simulink model "flight_sim"  (R2018b)
settings: Solver=FixedStepAuto  StartTime=0.0  StopTime=10  FixedStep=1.5  RelTol=1e-3
libraries: simulink x2, simulink_extras x1
settings Model: Creator=User  LastModifiedBy=Танечка
settings DebuggingCC: LibraryContextMissingDiagnostic=none
settings SFSimCC: SimUseLocalCustomCode=off
settings RTWCC: RTWUseLocalCustomCode=off

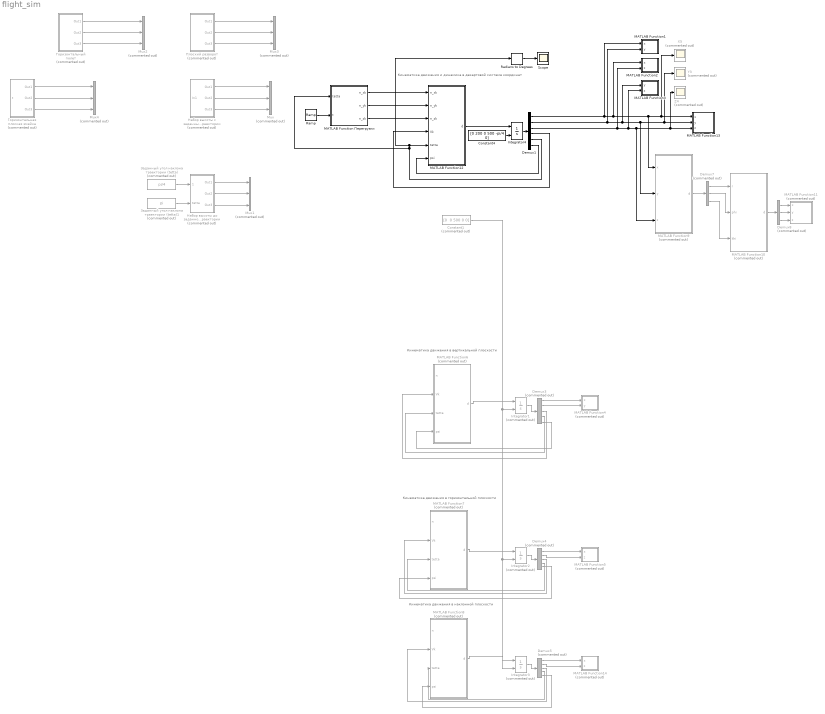
== system flight_sim ==
  note: Кинематика движения и динамика в декартовой системе координат
  note: Кинематика движения в вертикальной плоскости
  note: Кинематика движения в горизонтальной плоскости
  note: Кинематика движения в наклонной плоскости
  Constant1 : Constant  Commented=on  Value="[0  0 500 0 0]"
  Constant4 : Constant  Value=[0 200 0 500 -pi/4 0]
  Demux1 : Demux  Outputs=6
  Demux3 : Demux  Commented=on  Outputs=5
  Demux4 : Demux  Commented=on  Outputs=5
  Demux5 : Demux  Commented=on  Outputs=5
  Demux7 : Demux  Commented=on  Outputs=3
  Demux8 : Demux  Commented=on  Outputs=3
  Integrator1 : Integrator  Commented=on  InitialConditionSource=external
  Integrator2 : Integrator  Commented=on  InitialConditionSource=external
  Integrator3 : Integrator  Commented=on  InitialConditionSource=external
  Integrator4 : Integrator  InitialConditionSource=external
  MATLAB Function Перегрузки : MATLAB Function  TreatAsAtomicUnit=on
  MATLAB Function1 : MATLAB Function  TreatAsAtomicUnit=on
  MATLAB Function10 : MATLAB Function  Commented=on  TreatAsAtomicUnit=on
  MATLAB Function11 : MATLAB Function  Commented=on  TreatAsAtomicUnit=on
  MATLAB Function12 : MATLAB Function  TreatAsAtomicUnit=on
  MATLAB Function13 : MATLAB Function  TreatAsAtomicUnit=on
  MATLAB Function14 : MATLAB Function  Commented=on  TreatAsAtomicUnit=on
  MATLAB Function2 : MATLAB Function  TreatAsAtomicUnit=on
  MATLAB Function3 : MATLAB Function  TreatAsAtomicUnit=on
  MATLAB Function4 : MATLAB Function  Commented=on  TreatAsAtomicUnit=on
  MATLAB Function5 : MATLAB Function  Commented=on  TreatAsAtomicUnit=on
  MATLAB Function6 : MATLAB Function  Commented=on  TreatAsAtomicUnit=on
  MATLAB Function7 : MATLAB Function  Commented=on  TreatAsAtomicUnit=on
  MATLAB Function8 : MATLAB Function  Commented=on  TreatAsAtomicUnit=on
  MATLAB Function9 : MATLAB Function  Commented=on  TreatAsAtomicUnit=on
  Mux{,1..4} (5 alike) : Mux  Commented=on  Inputs=3
  Radians to Degrees : simulink_extras/Transformations/Radians to Degrees
  Ramp : simulink/Sources/Ramp  slope=1  start=0  InitialOutput=0
  Scope : Scope
  X5 : Scope  Commented=on
  Y3 : Scope  Commented=on
  Z4 : Scope  Commented=on
  Горизонтальная плоская змейка : Subsystem  Commented=on
  Горизонтальный полет : Subsystem  Commented=on
  Заданный угол наклона траектории (tetta) : Constant  Commented=on  Value=pi/4
  Заданный угол наклона траектории (tetta)1 : Constant  Commented=on  Value=pi
  Набор высоты до заданного угла наклона траектории : Subsystem  Commented=on
  "Набор высоты с заданным углом наклона траектории " : Subsystem  Commented=on
  Плоский разворот : Subsystem  Commented=on
  wires:
  Demux1/3 -> MATLAB Function2/2(z), MATLAB Function3/2(z), MATLAB Function9/3(z), MATLAB Function13/3(z), Z4/1
  Demux7/3 -> MATLAB Function10/3(khi)
  Demux7/2 -> MATLAB Function10/2(phi)
  Demux1/1 -> MATLAB Function1/1(x), MATLAB Function2/1(x), MATLAB Function9/1(x), X5/1, MATLAB Function13/1(x)
  Constant4/1 -> Integrator4/2
  MATLAB Function9/1(d) -> Demux7/1
  Demux1/5 -> MATLAB Function Перегрузки/1(tetta), MATLAB Function12/5(tetta), Radians to Degrees/1
  MATLAB Function10/1(d) -> Demux8/1
  Demux1/4 -> MATLAB Function12/4(Vk)
  Demux7/1 -> MATLAB Function10/1(r)
  Demux1/6 -> MATLAB Function12/6(psi)
  Integrator3/1 -> Demux5/1
  Demux3/2 -> MATLAB Function4/2(y)
  Constant1/1 -> Integrator1/2, Integrator3/2, Integrator2/2
  Integrator1/1 -> Demux3/1
  Demux5/2 -> MATLAB Function14/2(z)
  MATLAB Function6/1(d) -> Integrator1/1
  MATLAB Function8/1(d) -> Integrator3/1
  Demux5/1 -> MATLAB Function14/1(x)
  Demux4/2 -> MATLAB Function5/2(z)
  MATLAB Function7/1(d) -> Integrator2/1
  Integrator2/1 -> Demux4/1
  Demux4/1 -> MATLAB Function5/1(x)
  Demux3/1 -> MATLAB Function4/1(x)
  Demux3/3 -> MATLAB Function6/2(Vk)
  Demux3/4 -> MATLAB Function6/3(tetta)
  Demux3/5 -> MATLAB Function6/4(psi)
  Demux4/3 -> MATLAB Function7/2(Vk)
  Demux4/4 -> MATLAB Function7/3(tetta)
  Demux4/5 -> MATLAB Function7/4(psi)
  Demux5/3 -> MATLAB Function8/2(Vk)
  Demux5/4 -> MATLAB Function8/3(tetta)
  Demux5/5 -> MATLAB Function8/4(psi)
  Demux8/1 -> MATLAB Function11/1(x)
  Demux8/2 -> MATLAB Function11/2(y)
  Demux8/3 -> MATLAB Function11/3(z)
  MATLAB Function12/1(d) -> Integrator4/1
  Integrator4/1 -> Demux1/1
  Demux1/2 -> MATLAB Function1/2(y), MATLAB Function3/1(y), Y3/1, MATLAB Function13/2(y), MATLAB Function9/2(y)
  "Набор высоты с заданным углом наклона траектории "/1(Out1) -> Mux/1
  "Набор высоты с заданным углом наклона траектории "/2(Out2) -> Mux/2
  "Набор высоты с заданным углом наклона траектории "/3(Out3) -> Mux/3
  Заданный угол наклона траектории (tetta)/1 -> Набор высоты до заданного угла наклона траектории/1(tetta заданноне)
  Набор высоты до заданного угла наклона траектории/1(Out1) -> Mux1/1
  Набор высоты до заданного угла наклона траектории/2(Out2) -> Mux1/2
  Набор высоты до заданного угла наклона траектории/3(Out3) -> Mux1/3
  Заданный угол наклона траектории (tetta)1/1 -> Набор высоты до заданного угла наклона траектории/2(tetta)
  Горизонтальный полет/3(Out3) -> Mux2/3
  Горизонтальный полет/2(Out2) -> Mux2/2
  Горизонтальный полет/1(Out1) -> Mux2/1
  Плоский разворот/1(Out1) -> Mux3/1
  Плоский разворот/2(Out2) -> Mux3/2
  Плоский разворот/3(Out3) -> Mux3/3
  Горизонтальная плоская змейка/3(Out3) -> Mux4/3
  Горизонтальная плоская змейка/2(Out2) -> Mux4/2
  Горизонтальная плоская змейка/1(Out1) -> Mux4/1
  MATLAB Function Перегрузки/1(n_xk) -> MATLAB Function12/1(n_xk)
  MATLAB Function Перегрузки/2(n_yk) -> MATLAB Function12/2(n_yk)
  MATLAB Function Перегрузки/3(n_zk) -> MATLAB Function12/3(n_zk)
  Ramp/1 -> MATLAB Function Перегрузки/2(t)
  Radians to Degrees/1 -> Scope/1

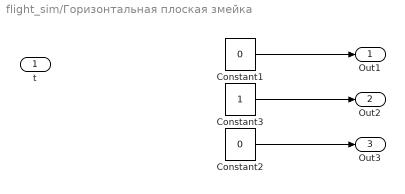
== system flight_sim/Горизонтальная плоская змейка ==
  t : Inport
  Constant1 : Constant  Value=0
  Constant2 : Constant  Value=0
  Constant3 : Constant
  Out1 : Outport
  Out2 : Outport  Port=2
  Out3 : Outport  Port=3
  wires:
  Constant2/1 -> Out3/1
  Constant3/1 -> Out2/1
  Constant1/1 -> Out1/1

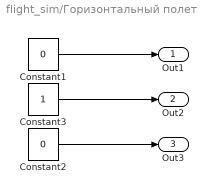
== system flight_sim/Горизонтальный полет ==
  Constant1 : Constant  Value=0
  Constant2 : Constant  Value=0
  Constant3 : Constant
  Out1 : Outport
  Out2 : Outport  Port=2
  Out3 : Outport  Port=3
  wires:
  Constant2/1 -> Out3/1
  Constant3/1 -> Out2/1
  Constant1/1 -> Out1/1

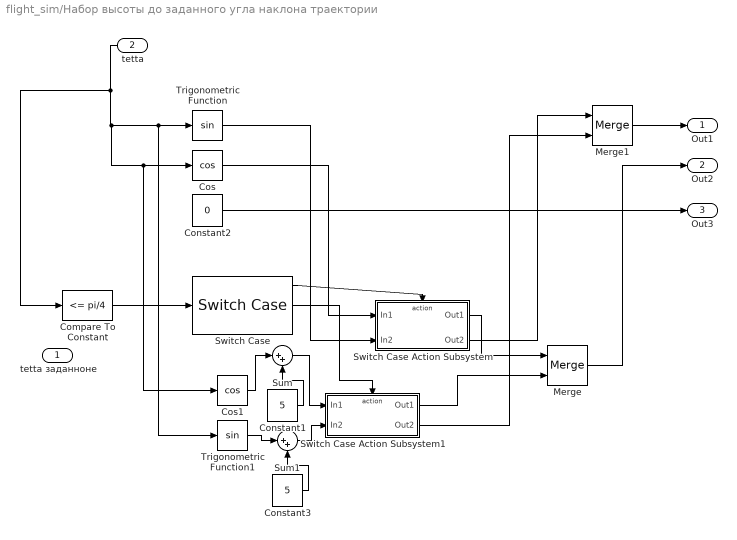
== system flight_sim/Набор высоты до заданного угла наклона траектории ==
  tetta заданноне : Inport
  tetta : Inport  Port=2
  Compare To Constant : simulink/Logic and Bit Operations/Compare To Constant  relop=<=  const=pi/4  OutDataTypeStr=uint8
  Constant1 : Constant  Value=5
  Constant2 : Constant  Value=0
  Constant3 : Constant  Value=5
  Cos : Trigonometry  Operator=cos
  Cos1 : Trigonometry  Operator=cos
  Merge : Merge
  Merge1 : Merge
  Sum : Sum  Inputs=|++
  Sum1 : Sum  Inputs=|++
  Switch Case : SwitchCase  CaseConditions={0,1}
  Switch Case Action Subsystem : Subsystem  TreatAsAtomicUnit=on
  Switch Case Action Subsystem1 : Subsystem  TreatAsAtomicUnit=on
  Trigonometric Function : Trigonometry
  Trigonometric Function1 : Trigonometry
  Out1 : Outport
  Out2 : Outport  Port=2
  Out3 : Outport  Port=3
  wires:
  Constant2/1 -> Out3/1
  Switch Case/1 -> Switch Case Action Subsystem/Action
  Switch Case/2 -> Switch Case Action Subsystem1/Action
  Switch Case Action Subsystem/1(Out1) -> Merge/1
  Switch Case Action Subsystem1/1(Out1) -> Merge/2
  Merge/1 -> Out2/1
  Cos/1 -> Switch Case Action Subsystem/1(In1)
  Cos1/1 -> Sum/1
  Compare To Constant/1 -> Switch Case/1
  Merge1/1 -> Out1/1
  Switch Case Action Subsystem/2(Out2) -> Merge1/1
  Switch Case Action Subsystem1/2(Out2) -> Merge1/2
  Trigonometric Function/1 -> Switch Case Action Subsystem/2(In2)
  tetta/1 -> Trigonometric Function1/1, Trigonometric Function/1, Cos/1, Cos1/1, Compare To Constant/1
  Sum/1 -> Switch Case Action Subsystem1/1(In1)
  Constant1/1 -> Sum/2
  Constant3/1 -> Sum1/2
  Trigonometric Function1/1 -> Sum1/1
  Sum1/1 -> Switch Case Action Subsystem1/2(In2)

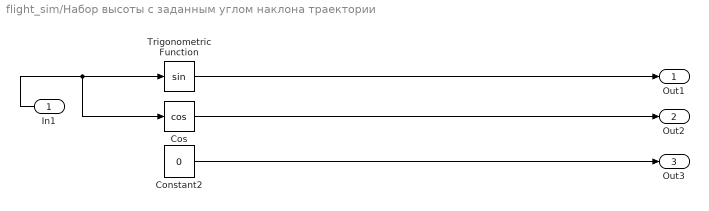
== system flight_sim/Набор высоты с заданным углом наклона траектории  ==
  In1 : Inport
  Constant2 : Constant  Value=0
  Cos : Trigonometry  Operator=cos
  Trigonometric Function : Trigonometry
  Out1 : Outport
  Out2 : Outport  Port=2
  Out3 : Outport  Port=3
  wires:
  Cos/1 -> Out2/1
  Constant2/1 -> Out3/1
  Trigonometric Function/1 -> Out1/1
  In1/1 -> Trigonometric Function/1, Cos/1

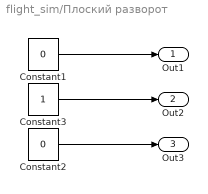
== system flight_sim/Плоский разворот ==
  Constant1 : Constant  Value=0
  Constant2 : Constant  Value=0
  Constant3 : Constant
  Out1 : Outport
  Out2 : Outport  Port=2
  Out3 : Outport  Port=3
  wires:
  Constant1/1 -> Out1/1
  Constant3/1 -> Out2/1
  Constant2/1 -> Out3/1

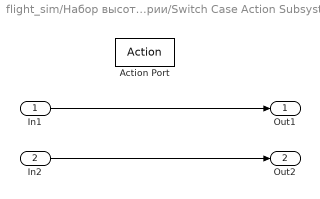
== system flight_sim/Набор высоты до заданного угла наклона траектории/Switch Case Action Subsystem ==
  In1 : Inport
  In2 : Inport  Port=2
  Action Port : ActionPort  ActionType=case
  Out1 : Outport
  Out2 : Outport  Port=2
  wires:
  In1/1 -> Out1/1
  In2/1 -> Out2/1

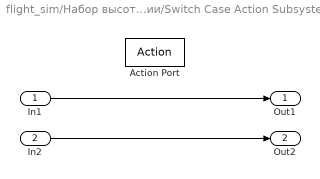
== system flight_sim/Набор высоты до заданного угла наклона траектории/Switch Case Action Subsystem1 ==
  In1 : Inport
  In2 : Inport  Port=2
  Action Port : ActionPort  ActionType=case
  Out1 : Outport
  Out2 : Outport  Port=2
  wires:
  In1/1 -> Out1/1
  In2/1 -> Out2/1

== matlab function flight_sim/MATLAB Function1 ==
  data: x input; y input
function plot2d(x,y)

figure(1);
plot(x,y,'ob');
hold on;

grid on;

xlabel('X');
ylabel('Y');
end

== matlab function flight_sim/MATLAB Function2 ==
  data: x input; z input
function plot2d(x,z)

figure(2);
plot(x,z,'ob');
hold on;

grid on;
xlabel('X');
ylabel('Z');
end

== matlab function flight_sim/MATLAB Function3 ==
  data: y input; z input
function plot2d(y,z)

figure(3);
plot(y,z,'ob');
hold on;

grid on;
xlabel('Y');
ylabel('Z');
end

== matlab function flight_sim/MATLAB Function6 ==
  data: n input; Vk input; d output; tetta input; psi input
function d  = diff(n,Vk,tetta,psi)

g = 9.81;
n_xk = n(1);
n_yk = n(2);
n_zk = n(3);

% Траекторного движения в вертикальной плоскости

dxg = Vk*cos(tetta)*cos(psi);      %xg
dyg = Vk*sin(tetta);               %yg

% Динамика траекторного движения
dVk    = g*(n_xk - sin(tetta));
dtetta = (g/Vk)*(n_yk - cos(tetta));
dpsi   = -(g*n_zk)/(Vk*cos(tetta));

d = [dxg dyg dVk dtetta dpsi];

end

== matlab function flight_sim/MATLAB Function14 ==
  data: x input; z input
function plot2d(x,z)

figure(7);
plot(x,z,'ob');
hold on;

grid on;
title('Движение в наклонной плоскости');
xlabel('X');
ylabel('Z');
end

== matlab function flight_sim/MATLAB Function4 ==
  data: x input; y input
function plot2d(x,y)

figure(5);
plot(x,y,'ob');
hold on;

grid on;
title('Движение в вертикальной плоскости');
xlabel('X');
ylabel('Y');
end

== matlab function flight_sim/MATLAB Function7 ==
  data: n input; Vk input; d output; tetta input; psi input
function d  = diff(n, Vk,tetta,psi)

g = 9.81;
n_xk = n(1);
n_yk = n(2);
n_zk = n(3);

% Траекторного движения в горизонтальной плоскости

dxg = Vk*cos(tetta)*cos(psi);      %xg
dzg = -Vk*cos(tetta)*sin(psi);     %zg

% Динамика траекторного движения
dVk    = g*(n_xk - sin(tetta));
dtetta = (g/Vk)*(n_yk - cos(tetta));
dpsi   = -(g*n_zk)/(Vk*cos(tetta));

d = [dxg dzg dVk dtetta dpsi];

end

== matlab function flight_sim/MATLAB Function8 ==
  data: n input; Vk input; d output; tetta input; psi input
function d  = diff(n, Vk,tetta,psi)

g = 9.81;
n_xk = n(1);
n_yk = n(2);
n_zk = n(3);


% Траекторного движения в наклонная плоскости

dxg = Vk*cos(psi);     %xg
dzg = -Vk*sin(psi);    %zg

% Динамика траекторного движения
dVk    = g*(n_xk - sin(tetta));
dtetta = (g/Vk)*(n_yk - cos(tetta));
dpsi   = -(g*n_zk)/(Vk*cos(tetta));

d = [dxg dzg dVk dtetta dpsi];
end

== matlab function flight_sim/MATLAB Function10 ==
  data: r input; d output; phi input; khi input
function d  = diff(r, phi, khi)

% Из сферической системе координат в декартову

dx = r*cos(phi)*cos(khi);
dy = r*sin(phi);             
dz = -r*cos(phi)*sin(khi);     

d = [dx dy dz];

end

== matlab function flight_sim/MATLAB Function11 ==
  data: x input; y input; z input
function plot3d(x,y, z)

figure(2);
plot3(x,z,y,'ob');
hold on;

grid on;

end

== matlab function flight_sim/MATLAB Function12 ==
  data: n_xk input; n_yk input; n_zk input; Vk input; d output; tetta input; psi input
function d  = diff(n_xk, n_yk, n_zk, Vk,tetta,psi)

% n_xk = n(1);
% n_yk = n(2);
% n_zk = n(3);

% tetta = deg2rad(tetta);
% psi   = deg2rad(psi);
g = 9.81;

% Кинематика траекторного движения
dxg = Vk*cos(tetta)*cos(psi);      %xg
dyg = Vk*sin(tetta);               %yg
dzg = -Vk*cos(tetta)*sin(psi);     %zg


% % Динамика траекторного движения
dVk    = g*(n_xk - sin(tetta));
dtetta = (g/Vk)*(n_yk - cos(tetta));
dpsi   = -(g*n_zk)/(Vk*cos(tetta));

d = [dxg dyg dzg dVk dtetta dpsi];
end

== matlab function flight_sim/MATLAB Function13 ==
  data: x input; y input; z input
function plot3d(x,y, z)

figure(4);
plot3(x,z,y,'ob');
hold on;

grid on;
xlabel('X');
ylabel('Z');
zlabel('Y');

end

== matlab function flight_sim/MATLAB Function9 ==
  data: x input; d output; y input; z input
function d  = diff(x, y, z)


% Кинематика в сферической системе координат

dr   = sqrt(x^2 + y^2 + z^2);
dphi = atan(y/(sqrt(x^2 + z^2)));             
dkhi = acos(x/(sqrt(x^2 + z^2)));     

d = [dr dphi dkhi];

end

== matlab function flight_sim/MATLAB Function5 ==
  data: x input; z input
function plot2d(x,z)

figure(6);
plot(x,z,'ob');
hold on;

grid on;
title('Движение в горизонтальной плоскости');
xlabel('X');
ylabel('Z');
end

== matlab function flight_sim/MATLAB Function Перегрузки ==
  data: tetta input; n_xk output; n_yk output; n_zk output; t input
function [n_xk, n_yk, n_zk]  = fcn(tetta, t)

% Равномерный прямолинейный горизонтальный полет:
% Начальные значения [0 0 0 500 0 0]


% n_xk = 0;
% n_yk = 1;
% n_zk = 0;

% Равномерный прямолинейный набор высоты с заданным углом наклона траектории:
% Начальные значения [0 0 0 500 pi/4 0]

% n_xk = sin(tetta);
% n_yk = cos(tetta);
% n_zk = 0;


% Равномерное прямолинейное снижение с заданным углом наклона траектории:
% Начальные значения [0 500 0 500 -pi/4 0]

n_xk = sin(tetta);
n_yk = cos(tetta);
n_zk = 0;



% Полет до заданного угла наклона траектории
% Начальные значения [0 0 0 500 pi/10 0]

% tetta_z = pi/4; % заданный угол наклона траектории
% 
% disp([tetta_z tetta]) 
% 
% if tetta <= tetta_z
%     n_xk = sin(tetta) + 1;
%     n_yk = cos(tetta) + 1;
%     n_zk = 0;
% else 
%     n_xk = sin(tetta);
%     n_yk = cos(tetta);
%     n_zk = 0;
% end



% Горизонтальный разворот с различными радиусами с постоянной скоростью
% Начальные значения [0 0 0 500 0 pi/6]

% n_xk=0;
% n_yk=1;
% n_zk=1;


% % Горизонтальная плоская змейка
% 
% n_xk = sin(tetta);
% n_yk = cos(tetta);
% n_zk = -cos(t);


% Вертикальная плоская змейка
% 
% n_xk = sin(tetta);
% n_yk = cos(tetta) + 10*cos(t);
% n_zk = 0;


% Пространственная змейка

% n_xk = sin(tetta);
% n_yk = cos(tetta) + 10*cos(t);
% n_zk = -cos(t)*cos(tetta);%чтобы устранить cos(tetta) в знаменателе


% n = [n_xk n_yk n_zk];
